simulink model "Mobile_Robot_Desired_Point"  (R2023a)
settings: Solver=VariableStepAuto  StartTime=0.0  StopTime=10  RelTol=1e-3
settings Model: Creator=pritesh.patel  LastModifiedBy=pritesh.patel

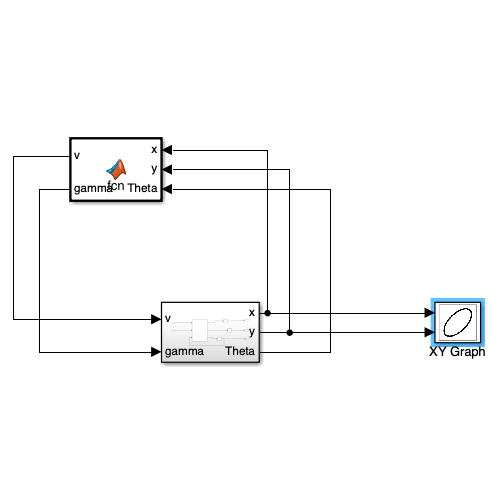
[thumbnail: Simulink's stored preview of the top-level diagram]
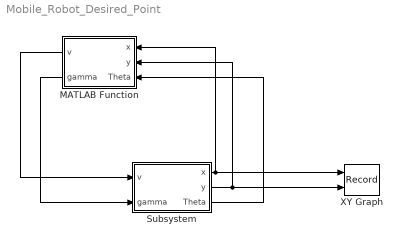
== system Mobile_Robot_Desired_Point ==
  MATLAB Function : MATLAB Function  TreatAsAtomicUnit=on
  Subsystem : Subsystem
  XY Graph : Record  FileSettingsInternal="{\"entries\":[{\"content\":{\"excelSettings\":{\"content\":{},\"type\":\"Streamout.ExcelSettings\"}},\"type\":\"Streamout.FileSettingStorage\",\"uuid\":\"\"}],\"packageUris\":[\"http:\\/\\/schema.mathworks.com\\/mf0\\/streamout_blocks\\/R2020a\"],\"version\":\"1.0\"}"  Layout=[1 1]  SignalsInternal="{\"entries\":[{\"content\":{\"signals\":[{\"content\":{\"blockPath\":[],\"dimensions\":[1],\"domain\":\"\",\"lineColor\":\"#a2142f\",\"plots\":[1],\"port\":1,\"sid\":[\"\"],\"signalID\":1247,\"signalName\":\"Subsystem:1\"},\"type\":\"RecordBlkView.Signal\",\"uuid\":\"\"},{\"content\":{\"blockPath\":[],\"dimensions\":[1],\"domain\":\"\",\"lineColor\":\"#139fff\",\"plots\":[1],\"port\":2,\"sid\":[\"\"],\"signalID\":1251,\"signalName\":\"Subsystem:2\"},\"type\":\"RecordBlkView.Signal\",\"uuid\":\"\"}]},\"type\":\"RecordBlkView.InputSignals\",\"uuid\":\"\"}],\"packageUris\":[\"http:\\/\\/schema.mathworks.com\\/mf0\\/streamout_blocks\\/R2020a\"],\"version\":\"1.0\"}"  VisualizationBindings="{\"xyplotplugin\":{\"info\":[{\"series\":[],\"subplotID\":1}]}}"  CompatibilityTag=XY
  wires:
  MATLAB Function/2(gamma) -> Subsystem/2(gamma)
  Subsystem/1(x) -> XY Graph/1, MATLAB Function/1(x)
  Subsystem/2(y) -> XY Graph/2, MATLAB Function/2(y)
  Subsystem/3(Theta) -> MATLAB Function/3(Theta)
  MATLAB Function/1(v) -> Subsystem/1(v)

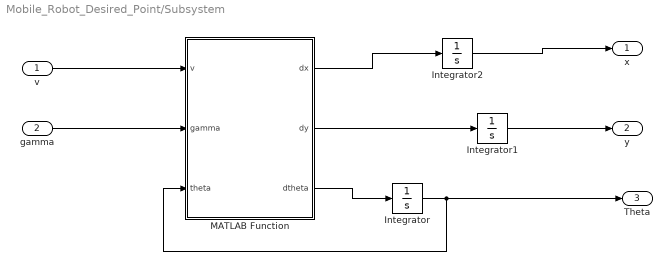
== system Mobile_Robot_Desired_Point/Subsystem ==
  v : Inport
  gamma : Inport  Port=2
  Integrator : Integrator  InitialCondition=pi/2
  Integrator1 : Integrator
  Integrator2 : Integrator
  MATLAB Function : MATLAB Function  TreatAsAtomicUnit=on
  x : Outport
  y : Outport  Port=2
  Theta : Outport  Port=3
  wires:
  Integrator1/1 -> y/1
  Integrator/1 -> Theta/1, MATLAB Function/3(theta)
  MATLAB Function/3(dtheta) -> Integrator/1
  Integrator2/1 -> x/1
  MATLAB Function/2(dy) -> Integrator1/1
  MATLAB Function/1(dx) -> Integrator2/1
  v/1 -> MATLAB Function/1(v)
  gamma/1 -> MATLAB Function/2(gamma)

== matlab function Mobile_Robot_Desired_Point/MATLAB Function ==
  data: x input; v output; y input; gamma output; Theta input
function [v, gamma] = fcn(x, y, Theta)
    % Desired position
    x_d = 5;
    y_d = 3;
    
    % Gain for velocity
    Kv = 0.5;
    
    % Gain for steering angle
    Kh = 1;
    
    % Calculate the distance to the desired position
    distance = sqrt((x_d - x)^2 + (y_d - y)^2);
    
    % Calculate the velocity input
    v = Kv * distance;
    
    % Calculate the desired angle using atan2 to avoid division by zero and handle all quadrants
    Theta_d = atan2(y_d - y, x_d - x);
    
    % Calculate the steering angle
    gamma = Kh * (Theta_d - Theta);
end

== matlab function Mobile_Robot_Desired_Point/Subsystem/MATLAB Function ==
  data: v input; gamma input; theta input; dx output; dy output; dtheta output
function [dx, dy, dtheta] = fcn(v, gamma, theta)
    % FCN calculates the change in position and orientation of a robot
    % given its velocity, steering angle, and current orientation.
    %
    % Inputs:
    %   v      - Velocity of the robot
    %   gamma  - Steering angle of the robot (in radians)
    %   theta  - Current orientation (heading angle) of the robot (in radians)
    %
    % Outputs:
    %   dx     - Change in x-coordinate of the robot
    %   dy     - Change in y-coordinate of the robot
    %   dtheta - Change in orientation of the robot
    
    % Wheelbase of the robot (distance between front and rear axles)
    L = 2;
    
    % Calculate the change in x-coordinate
    dx = v * cos(theta);
    
    % Calculate the change in y-coordinate
    dy = v * sin(theta);
    
    % Calculate the change in orientation
    dtheta = (v / L) * tan(gamma);
end
